simulink model "sdrrFMReceiverSimulink_true_fm_demod"  (R2018b)
settings: Solver=FixedStepDiscrete  StartTime=0.0  StopTime=inf  RelTol=1e-3
PreLoadFcn:
  | fmRxParams = helperFMConfig;
InitFcn:
  | fmRxParams = helperFMConfig;
undefined symbols (not defined in the file): designMultirateFIR
libraries: dsparch4 x2, dspsnks4 x1, simulink x1, dspmlti4 x1, commsource2 x1, commanabbnd3 x1, sdrrlib x1
Description:
  | This model uses either captured signals, or receive signals in real time
  | using RTL-SDR radio or ADALM-PLUTO radio with Simulink(R) to perform FM
  | demodulation and mono decoding.
settings Model: Creator=The MathWorks, Inc.  LastModifiedBy=79301
settings DataIOCC: SaveFormat=Structure  SaveOutput=off  SignalLogging=off  DSMLogging=off  SaveTime=off
settings OptimizationCC: ExpressionDepthLimit=2147483647  EfficientMapNaN2IntZero=off  LifeSpan=inf  SimCompilerOptimization=on
settings DebuggingCC: UnderspecifiedInitializationDetection=Classic  MergeDetectMultiDrivingBlocksExec=none  SolverPrmCheckMsg=warning  InheritedTsInSrcMsg=none  MultiTaskCondExecSysMsg=none  ParameterPrecisionLossMsg=none  FcnCallInpInsideContextMsg=warning  AllowSymbolicDim=off  StateNameClashWarn=warning  LibraryContextMissingDiagnostic=none  SFUnexpectedBacktrackingDiag=warning  SFNoUnconditionalDefaultTransitionDiag=warning  SFExecutionAtInitializationDiag=none
settings HardwareCC: ProdBitPerPointer=32  ProdBitPerSizeT=32  ProdBitPerPtrDiffT=32  ProdLargestAtomicFloat=None  ProdIntDivRoundTo=Undefined  ProdEndianess=Unspecified  ProdWordSize=32  ProdHWDeviceType=32-bit Generic  TargetBitPerPointer=64  TargetBitPerSizeT=64  TargetBitPerPtrDiffT=64  TargetLongLongMode=on  TargetIntDivRoundTo=Zero  TargetEndianess=LittleEndian  TargetWordSize=64  TargetHWDeviceType=Generic->MATLAB Host Computer  ProdEqTarget=off
settings ModelReferenceCC: PropagateSignalLabelsOutOfModel=off
settings SFSimCC: SimIntegrity=off  SimUseLocalCustomCode=off
settings RTWCC: RTWUseLocalCustomCode=off
settings RTWCC: CustomSourceCode=|
  | #include <stdio.h>
  | #include <stdlib.h>
settings CodeAppCC: MaxIdLength=128  StateflowObjectComments=on
settings GRTTargetCC: TargetLangStandard=C89/C90 (ANSI)  GeneratePreprocessorConditionals=Disable all  CombineOutputUpdateFcns=off  GRTInterface=on
settings ConfigComp: CovMetricSettings=dw  CovHtmlReporting=on  CovSaveCumulativeToWorkspaceVar=on  CovSaveSingleToWorkspaceVar=on  CovExternalEMLEnable=off  CovSFcnEnable=off

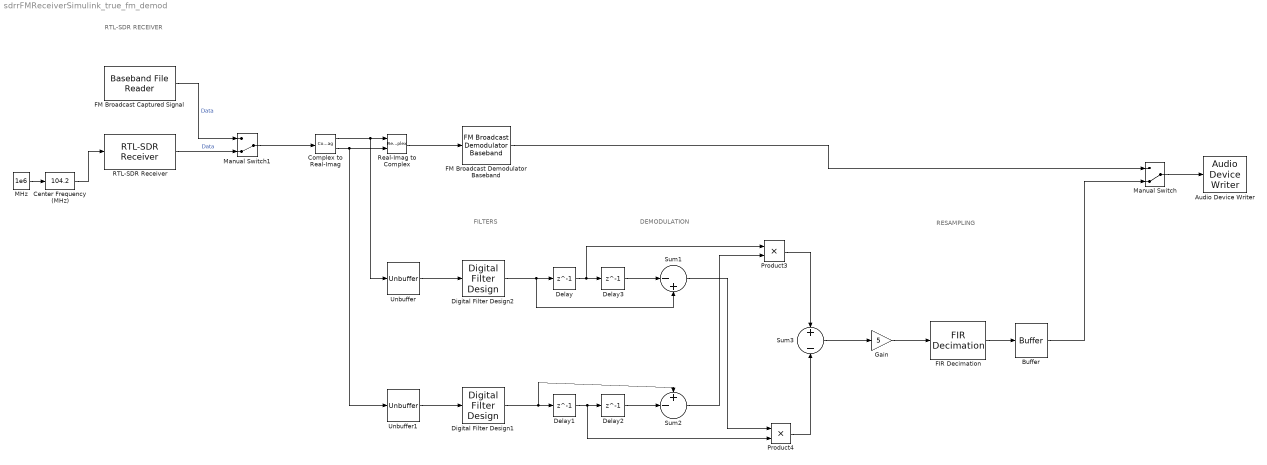
== system sdrrFMReceiverSimulink_true_fm_demod ==
  note: RESAMPLING
  note: DEMODULATION
  note: FILTERS
  note: RTL-SDR RECEIVER
  Audio Device Writer : dspsnks4/Audio Device Writer  Driver=DirectSound  Device=Default  InheritSampleRate=on  SampleRate=44100  BitDepth=16-bit integer  BufferSize=4096  NumBuffers=10  DefaultOutputChannelMapping=on  OutputChannelMapping=1:2  OutputNumUnderrunSamples=off  DriverIdx=1  DeviceWarnFlag=''
  Buffer : Buffer  N=768  OutputFrames=off
  Center Frequency (MHz) : simulink/Math Operations/Slider Gain  gain=104.2  low=87.9  high=107.9
  Complex to Real-Imag : ComplexToRealImag
  Delay{,1..3} (4 alike) : Delay  DelayLength=1  InitialCondition=0
  Digital Filter Design1 : dsparch4/Digital Filter Design  mwdsp_browser_bugfix_var=off
  Digital Filter Design2 : dsparch4/Digital Filter Design  mwdsp_browser_bugfix_var=off
  FIR Decimation : dspmlti4/FIR Decimation  FilterSource=Auto  h=designMultirateFIR(1,2)  D=5  filtStruct=Direct form  FilterObject=FDECIM  framing=Enforce single-rate processing  inputOffset=0  outputBufInitCond=0  roundingMode=Floor  overflowMode=off  firstCoeffDataTypeStr=Inherit: Same word length as input  firstCoeffMin=[]  firstCoeffMax=[]  firstCoeffLastDataTypeStr=Inherit: Same word length as input  outputDataTypeStr=Inherit: Same as accumulator  outputMin=[]  outputMax=[]  outputLastDataTypeStr=Inherit: Same as accumulator
  FM Broadcast Captured Signal : commsource2/Baseband File Reader  Filename=rbds_capture.bb  InheritSampleTimeFromFile=on  SampleTime=1  SamplesPerFrame=fmRxParams.FrontEndSamplesPerFrame  CyclicRepetition=on  FileEndOutputPort=off  SimulateUsing=Code generation
      settings: SourceProductName=Communications Toolbox  SourceProductBaseCode=CM
  FM Broadcast Demodulator Baseband : commanabbnd3/FM Broadcast Demodulator Baseband  SampleRate=fmRxParams.FrontEndSampleRate  FrequencyDeviation=fmRxParams.FrequencyDeviation  FilterTimeConstant=fmRxParams.FilterTimeConstant  AudioSampleRate=fmRxParams.AudioSampleRate  PlaySound=off  BufferSize=fmRxParams.BufferSize  Stereo=off  RBDS=off  RBDSSamplesPerSymbol=10  RBDSCostasLoop=off  SimulateUsing=Code generation
      settings: SourceProductName=Communications Toolbox  SourceProductBaseCode=CM
  Gain : Gain  Gain=5
  MHz : Constant  Value=1e6  VectorParams1D=off  SampleTime=-1  FramePeriod=-1
  Manual Switch : ManualSwitch  CurrentSetting=0
  Manual Switch1 : ManualSwitch  CurrentSetting=0
  Product3 : Product
  Product4 : Product
  RTL-SDR Receiver : sdrrlib/RTL-SDR Receiver  IPAddress=0  CenterFrequencySource=Input port  CenterFrequency=102.5e6  GainSource=AGC  Gain=0  ADCRate=fmRxParams.FrontEndSampleRate  FrequencyCorrection=0  LostSamplesOutputPort=off  LatencyOutputPort=off  OutputDataType=single  FrameLength=fmRxParams.FrontEndSamplesPerFrame  EnableBurstMode=off  NumFramesInBurst=20  sobjType=sdrr.internal.SDRRTLReceiverSL  dataUDPPort=-1  ctrlUDPPort=-1  subDeviceList=nosubdev  sdrBlockType=SDRBlockTypeSLT.SDRRxBlock  requester=UNUSED_BY_SFCN  sdrExecutionMode=SDRExecutionModeSLT.ExecModeHW  BypassUserLogic=off  DecimatorSelect=DDC decimator  SourceSelect=RF data  SineAmplitude=16000  EnableInternalClock=off  BypassIQBalance=off  IFBandwidth=40e6  ADCRateSource=Dialog  IntermediateFrequency=0  DecimationFactorSource=Dialog  DecimationFactor=512  RFFrequencyIsTunable=logical(1)  SampleTime=(fmRxParams.FrontEndSamplesPerFrame)/(fmRxParams.FrontEndSampleRate)  IFBandwidthSource=Dialog  SineFrequency=30000  BypassDCBlockingFilter=off  IntermediateFrequencySource=Dialog  IQBalanceCoefficients=64  SkipAllHardwareResetAndInitialization=off  EnableIQCalibrationTable=on  CacheIQCalibrationTable=off  EnableOffsetTuning=off  EnableRTLAGC=off  EnableTestMode=off  EnableTunerAGC=on  FrequencyCorrectionSource=Dialog  NumMLBuffers=128  NumUSBBuffers=16  RTLCrystalFrequency=28800000  TunerCrystalFrequency=28800000
      settings: SourceProductName=Communications System Toolbox Support Package for RTL-SDR Radio  SourceProductBaseCode=RTLSDR
  Real-Imag to Complex : RealImagToComplex
  Sum1 : Sum  Inputs=|-+
  Sum2 : Sum  Inputs=+-|
  Sum3 : Sum  Inputs=+|-
  Unbuffer : Unbuffer
  Unbuffer1 : Unbuffer
  wires:
  MHz/1 -> Center Frequency (MHz)/1
  Center Frequency (MHz)/1 -> RTL-SDR Receiver/1
  FM Broadcast Captured Signal/1 -> Manual Switch1/1  "Data"
  Manual Switch1/1 -> Complex to Real-Imag/1
  RTL-SDR Receiver/1 -> Manual Switch1/2  "Data"
  Real-Imag to Complex/1 -> FM Broadcast Demodulator Baseband/1
  Sum3/1 -> Gain/1
  Complex to Real-Imag/1 -> Unbuffer/1, Real-Imag to Complex/1
  Delay/1 -> Product3/1, Delay3/1
  Product4/1 -> Sum3/2
  Delay2/1 -> Sum2/2
  Delay3/1 -> Sum1/1
  Product3/1 -> Sum3/1
  Sum1/1 -> Product4/1
  Digital Filter Design1/1 -> Sum2/1, Delay1/1
  Delay1/1 -> Product4/2, Delay2/1
  Digital Filter Design2/1 -> Sum1/2, Delay/1
  Sum2/1 -> Product3/2
  Complex to Real-Imag/2 -> Unbuffer1/1, Real-Imag to Complex/2
  Unbuffer/1 -> Digital Filter Design2/1
  Unbuffer1/1 -> Digital Filter Design1/1
  Buffer/1 -> Manual Switch/2
  FIR Decimation/1 -> Buffer/1
  Gain/1 -> FIR Decimation/1
  Manual Switch/1 -> Audio Device Writer/1
  FM Broadcast Demodulator Baseband/1 -> Manual Switch/1
